simulink model "week2_problem_3"  (R2020b)
settings: Solver=VariableStepAuto  StartTime=0.0  StopTime=2  RelTol=1e-3
model workspace (MAT data in the model file):
  B = Simulink.Parameter
  B.Value = 50
  B.DataType = 'auto'
  B.Dimensions = [1 1]
  Kd = Simulink.Parameter
  Kd.Value = 484.0516
  Kd.DataType = 'auto'
  Kd.Dimensions = [1 1]
  Ki = Simulink.Parameter
  Ki.Value = 83.0917
  Ki.DataType = 'auto'
  Ki.Dimensions = [1 1]
  Kp = Simulink.Parameter
  Kp.Value = 495.0505
  Kp.DataType = 'auto'
  Kp.Dimensions = [1 1]
  M = Simulink.Parameter
  M.Value = 1000
  M.DataType = 'auto'
  M.Dimensions = [1 1]
settings Model: Creator=Yeshwanth  LastModifiedBy=Yeshwanth

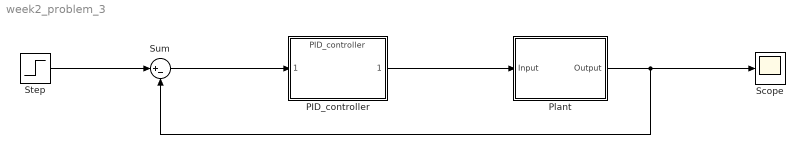
== system week2_problem_3 ==
  PID_controller : ModelReference  ModelNameDialog=PID_controller  SimulationMode=Normal  ModelReferenceVersion=1.6
  Plant : Subsystem
  Scope : Scope
  Step : Step  After=10  SampleTime=0
  Sum : Sum  Inputs=|+-
  wires:
  PID_controller/1 -> Plant/1(Input)
  Plant/1(Output) -> Scope/1, Sum/2
  Sum/1 -> PID_controller/1
  Step/1 -> Sum/1

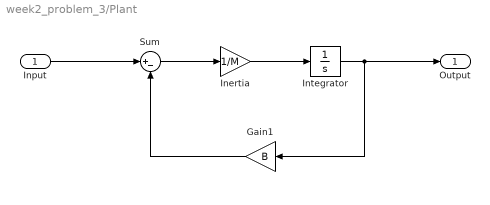
== system week2_problem_3/Plant ==
  Input : Inport
  Gain1 : Gain  Gain=B
  Inertia : Gain  Gain=1/M
  Integrator : Integrator
  Sum : Sum  Inputs=|+-
  Output : Outport
  wires:
  Sum/1 -> Inertia/1
  Integrator/1 -> Output/1, Gain1/1
  Gain1/1 -> Sum/2
  Inertia/1 -> Integrator/1
  Input/1 -> Sum/1
